simulink model "W14_Old_Town_cs"  (R2019a)
settings: Solver=ode5  StartTime=0.0  StopTime=inf  FixedStep=1/20  RelTol=1e-3
PreLoadFcn:
  | mbxruntime.callbacks.PreLoadFcn(bdroot);
PostLoadFcn:
  | mbxruntime.callbacks.PostLoadFcn(bdroot);
InitFcn:
  | mbxruntime.callbacks.InitFcn(bdroot);
StartFcn:
  | mbxruntime.callbacks.StartFcn(bdroot);
StopFcn:
  | mbxruntime.callbacks.StopFcn(bdroot);
model workspace: external: MAT-File .\W14_Old_Town_cs_hws.mat (data not in the file)
undefined symbols (not defined in the file or in its folder): DiscIntNeverNeededParam, InitImageOutputDir, mbxruntime, tabledata, W14_Old_Town_cs_420627b55bfa6657, W14_Old_Town_cs_65496e67f8744427, W14_Old_Town_cs_7675d4d8a4ff2559, W14_Old_Town_cs_7e35845ee4621ce0, W14_Old_Town_cs_873234be1b10e463, W14_Old_Town_cs_9ef39b80314364c8, W14_Old_Town_cs_a7463be4909f0caf, W14_Old_Town_cs_adbd81c42fc98a6f, W14_Old_Town_cs_Audi_A8_Sedan_1_Path_pathUniqueID, W14_Old_Town_cs_b1d069d1f3eacd72, W14_Old_Town_cs_Child_Regular_1_Path_pathUniqueID, W14_Old_Town_cs_Child_Regular_2_Path_pathUniqueID, W14_Old_Town_cs_Citroen_C3_Hatchback_1_Path_pathUniqueID, W14_Old_Town_cs_dbeb6fac3e8a4bef, W14_Old_Town_cs_fc5b0755bd4a98fc, W14_Old_Town_cs_Man_250_1_Path_pathUniqueID, W14_Old_Town_cs_Man_250_1_SpeedProfile_speedProfileUniqueID, W14_Old_Town_cs_Mazda_RX8_Coupe_1_Path_pathUniqueID
libraries: adeye_lib x38, simulink_extras x21, simulink x5, PreScanSimulinkLibrary x2, PreScanUsefulBlocks x1
(part 1 of 7)
CloseFcn:
  | mbxruntime.callbacks.CloseFcn(bdroot);
settings Model: Creator=PRESCAN  LastModifiedBy=adeye
settings DataIOCC: LimitDataPoints=on  SaveFormat=Array  SignalLoggingSaveFormat=ModelDataLogs  ReturnWorkspaceOutputs=off
settings OptimizationCC: DefaultParameterBehavior=Inlined  ExpressionDepthLimit=2147483647  InitFltsAndDblsToZero=on  LifeSpan=inf
settings DebuggingCC: SaveWithParameterizedLinksMsg=none  UnderspecifiedInitializationDetection=Classic  MergeDetectMultiDrivingBlocksExec=none  SignalResolutionControl=TryResolveAllWithWarning  MultiTaskDSMMsg=warning  MultiTaskCondExecSysMsg=none  FcnCallInpInsideContextMsg=warning  StateNameClashWarn=warning  SFUnexpectedBacktrackingDiag=warning  SFNoUnconditionalDefaultTransitionDiag=warning  SFExecutionAtInitializationDiag=none  ArithmeticOperatorsInVariantConditions=warning
settings HardwareCC: ProdBitPerPointer=32  ProdBitPerSizeT=32  ProdBitPerPtrDiffT=32  ProdLargestAtomicFloat=None  ProdIntDivRoundTo=Undefined  ProdEndianess=Unspecified  ProdWordSize=32  ProdHWDeviceType=32-bit Generic
settings ModelReferenceCC: UpdateModelReferenceTargets=IfOutOfDate  PropagateSignalLabelsOutOfModel=off
settings SFSimCC: SimUseLocalCustomCode=off  SimParseCustomCode=off
settings SFSimCC: SimCustomHeaderCode=|
  | #include "prescan.h"
  | #include "prescan_platform.h"
settings RTWCC: RTWUseLocalCustomCode=off
settings CodeAppCC: StateflowObjectComments=on
settings GRTTargetCC: TargetFcnLib=ansi_tfl_tmw.mat  TargetLangStandard=C89/C90 (ANSI)  GeneratePreprocessorConditionals=Disable all  CombineOutputUpdateFcns=off  GRTInterface=on
settings ConfigComp: CovMetricSettings=dw  CovHtmlReporting=on  CovSaveCumulativeToWorkspaceVar=on  CovSaveSingleToWorkspaceVar=on  CovExternalEMLEnable=off  CovSFcnEnable=off

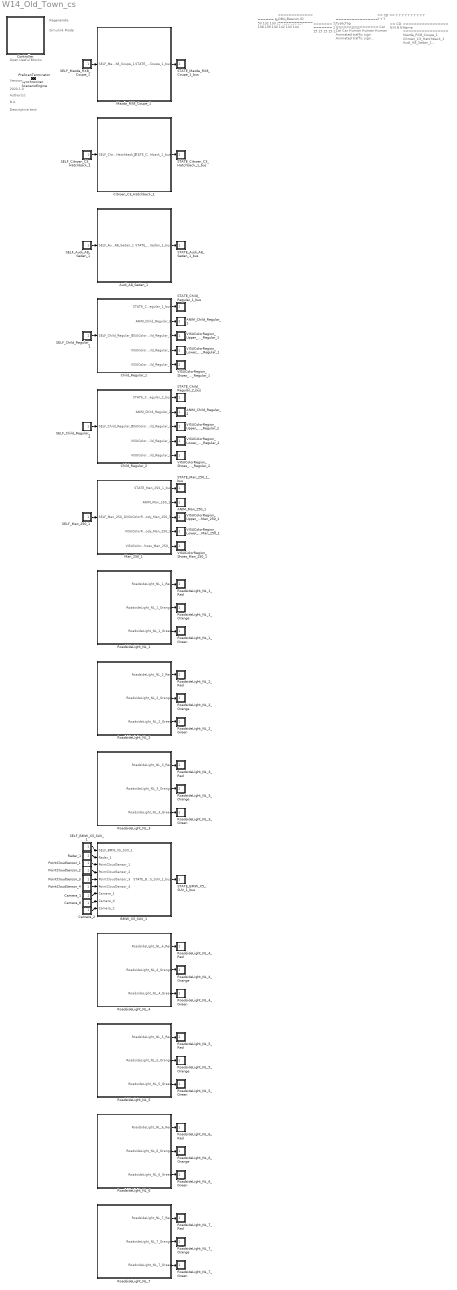
== system W14_Old_Town_cs ==
  note: Regenerate
  note: Simulink Mode
  note: Open Useful Blocks
  note: 2020.1.0
  note: Version:
  note: Author(s):
  note: N.A.
  note: Descriptive text:
  note: ======
      | Num ID
      | ======
      | 53
      | 132
      | 133
      | 134
      | 135
      | 136
      | 137
      | 138
      | 139
      | 140
      | 142
      | 143
      | 144
  note: =============
      | OBU-Beacon ID
      | =============
  note: =======
      | Type ID
      | =======
      | 1
      | 1
      | 1
      | 4
      | 4
      | 4
      | 15
      | 15
      | 15
      | 15
      | 15
      | 15
      | 15
  note: ================
      | Type Tag
      | ================
      | Car
      | Car
      | Car
      | Human
      | Human
      | Human
      | Animated traffic sign
      | Animated traffic sign
      | Animated traffic sign
      | Animated traffic sign
      | Animated traffic sign
      | Animated traffic sign
      | Animated traffic sign
  note: ==
      | SD
      | ==
      | Y
      | Y
      | Y
      | Y
      | Y
      | Y
      | Y
      | Y
      | Y
      | Y
      | Y
      | Y
      | Y
  note: ==
      | CD
      | ==
      | N
      | N
      | N
      | N
      | N
      | N
      | N
      | N
      | N
      | N
      | N
      | N
      | N
  note: =================
      | Name
      | =================
      | Mazda_RX8_Coupe_1
      | Citroen_C3_Hatchback_1
      | Audi_A8_Sedan_1
      | Child_Regular_1
      | Child_Regular_2
      | Man_250_1
      | RoadsideLight_NL_1
      | RoadsideLight_NL_2
      | RoadsideLight_NL_3
      | RoadsideLight_NL_4
      | RoadsideLight_NL_5
      | RoadsideLight_NL_6
      | RoadsideLight_NL_7
  ANIM_Child_Regular_1 : Subsystem  Tag=actuator/AnimationOutport  Priority=0  LoadFcn=load('PreScanAnimActuatorData.mat')  mask(PreScan Sink Block: State Animation){}
      mask help: The Human Animation port allows the human to walk, run or bend
      settings: OpenFcn=open_system([gcb '/Actuator'],'mask')
      mask Help: eval('openHelp(239)')
      mask Display: image(imread('HumanAnimated.jpg'))
  ANIM_Child_Regular_2 : Subsystem  Tag=actuator/AnimationOutport  Priority=0  LoadFcn=load('PreScanAnimActuatorData.mat')  mask(PreScan Sink Block: State Animation){}
      mask help: The Human Animation port allows the human to walk, run or bend
      settings: OpenFcn=open_system([gcb '/Actuator'],'mask')
      mask Help: eval('openHelp(239)')
      mask Display: image(imread('HumanAnimated.jpg'))
  ANIM_Man_250_1 : Subsystem  Tag=actuator/AnimationOutport  Priority=0  LoadFcn=load('PreScanAnimActuatorData.mat')  mask(PreScan Sink Block: State Animation){}
      mask help: The Human Animation port allows the human to walk, run or bend
      settings: OpenFcn=open_system([gcb '/Actuator'],'mask')
      mask Help: eval('openHelp(239)')
      mask Display: image(imread('HumanAnimated.jpg'))
  Audi_A8_Sedan_1 : Subsystem  Tag=WorldObjectSubSystem  InitFcn=UniqueId = '6579';
      mask init:
      | modelPath = GenericModelHelper.getGenericModelFilePath('ModelDepo','Vehicles\Audi_A8\Audi_A8.pgmb','e33fe1ddcf3e8ae97caccbc8f2fa74ac');imagePath = GenericModelHelper.getCompilationPicture(modelPath, 'Audi_A8_HighPoly.png');
      mask Display: image(imread(imagePath));color('white');text(0, 0, ' ID=133\n')
  BMW_X5_SUV_1 : Subsystem  Tag=WorldObjectSubSystem  InitFcn=|
      | UniqueId = '6361';
      | UniqueId = '6795';
      mask init:
      | modelPath = GenericModelHelper.getGenericModelFilePath('ModelDepo','Vehicles\BMW_X5\BMW_X5.pgmb','bfeb1c11467705ab888b3011684c848b');imagePath = GenericModelHelper.getCompilationPicture(modelPath, 'BMW_X5_HighPoly.png');
      mask Display: image(imread(imagePath));color('white');text(0, 0, ' ID=141\n')
  Camera_1 : Subsystem  Tag=sensor/Camera/CameraSensor  Priority=30  mask(PreScan Source Block: Camera Sensor){}
      mask help: The Camera Sensor provides a color or monochrome image.
      settings: OpenFcn=open_system([gcb '/Sensor'],'mask')
      mask Help: eval('openHelp(457)')
      mask Display: image(imread('CameraSensor.png'))
  Camera_2 : Subsystem  Tag=sensor/Camera/CameraSensor  Priority=30  mask(PreScan Source Block: Camera Sensor){}
      mask help: The Camera Sensor provides a color or monochrome image.
      settings: OpenFcn=open_system([gcb '/Sensor'],'mask')
      mask Help: eval('openHelp(457)')
      mask Display: image(imread('CameraSensor.png'))
  Camera_tl : Subsystem  Tag=sensor/Camera/CameraSensor  Priority=30  mask(PreScan Source Block: Camera Sensor){}
      mask help: The Camera Sensor provides a color or monochrome image.
      settings: OpenFcn=open_system([gcb '/Sensor'],'mask')
      mask Help: eval('openHelp(457)')
      mask Display: image(imread('CameraSensor.png'))
  Child_Regular_1 : Subsystem  Tag=WorldObjectSubSystem  InitFcn=UniqueId = '6584';
      mask init:
      | modelPath = GenericModelHelper.getGenericModelFilePath('ModelDepo','Humans\ChildRegular\Child_Regular.pgmb','0405fb6e1c51d7af34e60031bef9e83f');imagePath = GenericModelHelper.getCompilationPicture(modelPath, 'ChildRegular.png');
      mask Display: image(imread(imagePath));color('white');text(0, 0, ' ID=134\n')
  Child_Regular_2 : Subsystem  Tag=WorldObjectSubSystem  InitFcn=UniqueId = '6587';
      mask init: same as W14_Old_Town_cs/Child_Regular_1
      mask Display: image(imread(imagePath));color('white');text(0, 0, ' ID=135\n')
  Citroen_C3_Hatchback_1 : Subsystem  Tag=WorldObjectSubSystem  InitFcn=UniqueId = '6576';
      mask init:
      | modelPath = GenericModelHelper.getGenericModelFilePath('ModelDepo','Vehicles\Citroen_C3\Citroen_C3.pgmb','e804ced06d50dbfc6a2202ab3ad01b0c');imagePath = GenericModelHelper.getCompilationPicture(modelPath, 'Citroen_C3_HighPoly.png');
      mask Display: image(imread(imagePath));color('white');text(0, 0, ' ID=132\n')
  Controller : Subsystem  Description=8A3CD2955739A82C886C20AE3E253D78460D53180EE2C1B14CC08DF75A70BE77  Priority=-1  LoadFcn=load PreScanControllerData  mask(PreScan Simulation Controller){prescanversion='2020.1.0', ModelReferencing=off, TimeStep=1/20, ControlMode=0, PreScanExecutionMode=on, ControllerCount=0, ControllerIndex=0, ControllerOptions=''}
      mask prompts: prescanversion "PreScan Version"; ModelReferencing "Use Model Referencing"; TimeStep "Upload Period [s]"; ControlMode "Control Mode"; PreScanExecutionMode "Execution Mode"; ControllerCount "Controller Count"; ControllerIndex "Controller Index"; ControllerOptions "Controller Options"
      mask help:
      | Please do not remove this block from the compilation sheet,
      | as it connects the model to the PreScan environment.
      mask init:
      | model = bdroot(gcb);
      | ExperimentFile = mbxruntime.findExperimentFile(model,true); %relative path
      | 
      | [d1, d2, d3, prescandata] = prescan_Settings();
      | ModelDepo = fullfile(prescandata,'ModelDepo'); 
      | 
      | RTmode = mbxruntime.getRTMode(model);
      | 
      | SimulationMode = get_param(bdroot,'SimulationMode');
      | if strcmp(SimulationMode, 'rapid-accelerator')
      |     SimulationMode = 'external';
      | end
      | TargetName = get_param(bdroot,'SystemTargetFile');
      settings: ModelCloseFcn=assignin('base',['model_closed_' bdroot],true);
      mask Help: eval('openHelp(812)')
      mask Display: image(imread('prescanlogo.ico'))
  Man_250_1 : Subsystem  Tag=WorldObjectSubSystem  InitFcn=UniqueId = '6591';
      mask init:
      | modelPath = GenericModelHelper.getGenericModelFilePath('ModelDepo','Humans\Man_250\Man_250.pgmb','d552687b60780d871f7a0144e7f81878');imagePath = GenericModelHelper.getCompilationPicture(modelPath, 'Man_250.png');
      mask Display: image(imread(imagePath));color('white');text(0, 0, ' ID=136\n')
  Mazda_RX8_Coupe_1 : Subsystem  Tag=WorldObjectSubSystem  InitFcn=UniqueId = '6573';
      mask init:
      | modelPath = GenericModelHelper.getGenericModelFilePath('ModelDepo','Vehicles\Mazda_RX8\Mazda_RX8.pgmb','1e55a2e40efa576b7f4fb93bae35d605');imagePath = GenericModelHelper.getCompilationPicture(modelPath, 'Mazda_RX8_HighPoly.png');
      mask Display: image(imread(imagePath));color('white');text(0, 0, ' ID=53\n')
  PointCloudSensor_1 : Subsystem  Tag=sensor/PointCloudInport  Priority=30  mask(PreScan Source Block: Point Cloud Sensor){}
      mask help: The Point Cloud Sensor provides XYZ positions relative to the sensor
      settings: OpenFcn=open_system([gcb '/Sensor'],'mask')
      mask Help: eval('openHelp(6400)')
      mask Display: image(imread('PointCloudSensorSL.png'))
  PointCloudSensor_2 : Subsystem  Tag=sensor/PointCloudInport  Priority=30  mask(PreScan Source Block: Point Cloud Sensor){}
      mask help: The Point Cloud Sensor provides XYZ positions relative to the sensor
      settings: OpenFcn=open_system([gcb '/Sensor'],'mask')
      mask Help: eval('openHelp(6400)')
      mask Display: image(imread('PointCloudSensorSL.png'))
  PointCloudSensor_3 : Subsystem  Tag=sensor/PointCloudInport  Priority=30  mask(PreScan Source Block: Point Cloud Sensor){}
      mask help: The Point Cloud Sensor provides XYZ positions relative to the sensor
      settings: OpenFcn=open_system([gcb '/Sensor'],'mask')
      mask Help: eval('openHelp(6400)')
      mask Display: image(imread('PointCloudSensorSL.png'))
  PointCloudSensor_4 : Subsystem  Tag=sensor/PointCloudInport  Priority=30  mask(PreScan Source Block: Point Cloud Sensor){}
      mask help: The Point Cloud Sensor provides XYZ positions relative to the sensor
      settings: OpenFcn=open_system([gcb '/Sensor'],'mask')
      mask Help: eval('openHelp(6400)')
      mask Display: image(imread('PointCloudSensorSL.png'))
  PreScanTerminator : Subsystem  Tag=PreScanTerminator  Priority=999  LoadFcn=load PrescanTerminatorData  mask(PreScan Simulation Terminator){TimeStep=1/20}
      mask prompts: TimeStep "Upload Period [s]"
      mask help:
      | Please do not remove this block from the compilation sheet as it
      | connects the model to the PreScan environment.
      mask Help: eval('openHelp(812)')
      mask Display: image(imread('prescanlogo.ico'))
  Radar_1 : Subsystem  Tag=sensor/Radar  Priority=30  LoadFcn=load('PrescanScannerSensorData.mat');load('PrescanScannerSensorMessage.mat')  mask(PreScan Source Block: Radar Sensor){}
      mask help:
      | The Radar Sensor is a detailed sensor based on a physical radar
      | model that includes Antenna GAIN Maps (AGM) and atmospheric
      | attenuation.
      |
      | For more information, please click Help.
      settings: OpenFcn=open_system([gcb '/Sensor'],'mask')
      mask Help: eval('openHelp(1464)')
      mask Display: image(imread('Radar.png'))
  RoadsideLight_NL_1 : Subsystem  Tag=WorldObjectSubSystem  InitFcn=UniqueId = '6597';
      mask init:
      | modelPath = GenericModelHelper.getGenericModelFilePath('ModelDepo','AnimatedElements\TrafficLight_NL\Roadside\Roadside_NL.pgmb','2000fba5e1a6d0fba32e88146243c3cb');imagePath = GenericModelHelper.getCompilationPicture(modelPath, 'Roadside_NL.png');
      mask Display: image(imread(imagePath));color('white');text(0, 0, ' ID=137\n')
  RoadsideLight_NL_1_Green : Subsystem  Tag=actuator/Green  Priority=0  LoadFcn=load('PreScanVisuLightActuatorData');load('PrescanRPYData');load('PrescanXYZData');load('PreScanRGBData')  mask(PreScan Sink Block: VisuActiveLight){}
      mask help:
      | The VisuActiveLight block provides a way for detailed animation of Light Sources, such as the indicator, brake, fog and main lights of a vehicle, or a light post.
      |
      | For more information, please click Help.
      settings: OpenFcn=open_system([gcb '/Actuator'],'mask')
      mask Help: eval('openHelp(209)')
      mask Display: image(imread('HeadLight.png'))
  RoadsideLight_NL_1_Orange : Subsystem  Tag=actuator/Orange  Priority=0  LoadFcn=load('PreScanVisuLightActuatorData');load('PrescanRPYData');load('PrescanXYZData');load('PreScanRGBData')  mask(PreScan Sink Block: VisuActiveLight){}
      mask help:
      | The VisuActiveLight block provides a way for detailed animation of Light Sources, such as the indicator, brake, fog and main lights of a vehicle, or a light post.
      |
      | For more information, please click Help.
      settings: OpenFcn=open_system([gcb '/Actuator'],'mask')
      mask Help: eval('openHelp(209)')
      mask Display: image(imread('HeadLight.png'))
  RoadsideLight_NL_1_Red : Subsystem  Tag=actuator/Red  Priority=0  LoadFcn=load('PreScanVisuLightActuatorData');load('PrescanRPYData');load('PrescanXYZData');load('PreScanRGBData')  mask(PreScan Sink Block: VisuActiveLight){}
      mask help:
      | The VisuActiveLight block provides a way for detailed animation of Light Sources, such as the indicator, brake, fog and main lights of a vehicle, or a light post.
      |
      | For more information, please click Help.
      settings: OpenFcn=open_system([gcb '/Actuator'],'mask')
      mask Help: eval('openHelp(209)')
      mask Display: image(imread('HeadLight.png'))
  RoadsideLight_NL_2 : Subsystem  Tag=WorldObjectSubSystem  InitFcn=UniqueId = '6598';
      mask init: same as W14_Old_Town_cs/RoadsideLight_NL_1
      mask Display: image(imread(imagePath));color('white');text(0, 0, ' ID=138\n')
  RoadsideLight_NL_2_Green : Subsystem  Tag=actuator/Green  Priority=0  LoadFcn=load('PreScanVisuLightActuatorData');load('PrescanRPYData');load('PrescanXYZData');load('PreScanRGBData')  mask(PreScan Sink Block: VisuActiveLight){}
      mask help:
      | The VisuActiveLight block provides a way for detailed animation of Light Sources, such as the indicator, brake, fog and main lights of a vehicle, or a light post.
      |
      | For more information, please click Help.
      settings: OpenFcn=open_system([gcb '/Actuator'],'mask')
      mask Help: eval('openHelp(209)')
      mask Display: image(imread('HeadLight.png'))
  RoadsideLight_NL_2_Orange : Subsystem  Tag=actuator/Orange  Priority=0  LoadFcn=load('PreScanVisuLightActuatorData');load('PrescanRPYData');load('PrescanXYZData');load('PreScanRGBData')  mask(PreScan Sink Block: VisuActiveLight){}
      mask help:
      | The VisuActiveLight block provides a way for detailed animation of Light Sources, such as the indicator, brake, fog and main lights of a vehicle, or a light post.
      |
      | For more information, please click Help.
      settings: OpenFcn=open_system([gcb '/Actuator'],'mask')
      mask Help: eval('openHelp(209)')
      mask Display: image(imread('HeadLight.png'))
  RoadsideLight_NL_2_Red : Subsystem  Tag=actuator/Red  Priority=0  LoadFcn=load('PreScanVisuLightActuatorData');load('PrescanRPYData');load('PrescanXYZData');load('PreScanRGBData')  mask(PreScan Sink Block: VisuActiveLight){}
      mask help:
      | The VisuActiveLight block provides a way for detailed animation of Light Sources, such as the indicator, brake, fog and main lights of a vehicle, or a light post.
      |
      | For more information, please click Help.
      settings: OpenFcn=open_system([gcb '/Actuator'],'mask')
      mask Help: eval('openHelp(209)')
      mask Display: image(imread('HeadLight.png'))
  RoadsideLight_NL_3 : Subsystem  Tag=WorldObjectSubSystem  InitFcn=UniqueId = '6599';
      mask init: same as W14_Old_Town_cs/RoadsideLight_NL_1
      mask Display: image(imread(imagePath));color('white');text(0, 0, ' ID=139\n')
  RoadsideLight_NL_3_Green : Subsystem  Tag=actuator/Green  Priority=0  LoadFcn=load('PreScanVisuLightActuatorData');load('PrescanRPYData');load('PrescanXYZData');load('PreScanRGBData')  mask(PreScan Sink Block: VisuActiveLight){}
      mask help:
      | The VisuActiveLight block provides a way for detailed animation of Light Sources, such as the indicator, brake, fog and main lights of a vehicle, or a light post.
      |
      | For more information, please click Help.
      settings: OpenFcn=open_system([gcb '/Actuator'],'mask')
      mask Help: eval('openHelp(209)')
      mask Display: image(imread('HeadLight.png'))
  RoadsideLight_NL_3_Orange : Subsystem  Tag=actuator/Orange  Priority=0  LoadFcn=load('PreScanVisuLightActuatorData');load('PrescanRPYData');load('PrescanXYZData');load('PreScanRGBData')  mask(PreScan Sink Block: VisuActiveLight){}
      mask help:
      | The VisuActiveLight block provides a way for detailed animation of Light Sources, such as the indicator, brake, fog and main lights of a vehicle, or a light post.
      |
      | For more information, please click Help.
      settings: OpenFcn=open_system([gcb '/Actuator'],'mask')
      mask Help: eval('openHelp(209)')
      mask Display: image(imread('HeadLight.png'))
  RoadsideLight_NL_3_Red : Subsystem  Tag=actuator/Red  Priority=0  LoadFcn=load('PreScanVisuLightActuatorData');load('PrescanRPYData');load('PrescanXYZData');load('PreScanRGBData')  mask(PreScan Sink Block: VisuActiveLight){}
      mask help:
      | The VisuActiveLight block provides a way for detailed animation of Light Sources, such as the indicator, brake, fog and main lights of a vehicle, or a light post.
      |
      | For more information, please click Help.
      settings: OpenFcn=open_system([gcb '/Actuator'],'mask')
      mask Help: eval('openHelp(209)')
      mask Display: image(imread('HeadLight.png'))
  RoadsideLight_NL_4 : Subsystem  Tag=WorldObjectSubSystem  InitFcn=UniqueId = '6804';
      mask init: same as W14_Old_Town_cs/RoadsideLight_NL_1
      mask Display: image(imread(imagePath));color('white');text(0, 0, ' ID=140\n')
  RoadsideLight_NL_4_Green : Subsystem  Tag=actuator/Green  Priority=0  LoadFcn=load('PreScanVisuLightActuatorData');load('PrescanRPYData');load('PrescanXYZData');load('PreScanRGBData')  mask(PreScan Sink Block: VisuActiveLight){}
      mask help:
      | The VisuActiveLight block provides a way for detailed animation of Light Sources, such as the indicator, brake, fog and main lights of a vehicle, or a light post.
      |
      | For more information, please click Help.
      settings: OpenFcn=open_system([gcb '/Actuator'],'mask')
      mask Help: eval('openHelp(209)')
      mask Display: image(imread('HeadLight.png'))
  RoadsideLight_NL_4_Orange : Subsystem  Tag=actuator/Orange  Priority=0  LoadFcn=load('PreScanVisuLightActuatorData');load('PrescanRPYData');load('PrescanXYZData');load('PreScanRGBData')  mask(PreScan Sink Block: VisuActiveLight){}
      mask help:
      | The VisuActiveLight block provides a way for detailed animation of Light Sources, such as the indicator, brake, fog and main lights of a vehicle, or a light post.
      |
      | For more information, please click Help.
      settings: OpenFcn=open_system([gcb '/Actuator'],'mask')
      mask Help: eval('openHelp(209)')
      mask Display: image(imread('HeadLight.png'))
  RoadsideLight_NL_4_Red : Subsystem  Tag=actuator/Red  Priority=0  LoadFcn=load('PreScanVisuLightActuatorData');load('PrescanRPYData');load('PrescanXYZData');load('PreScanRGBData')  mask(PreScan Sink Block: VisuActiveLight){}
      mask help:
      | The VisuActiveLight block provides a way for detailed animation of Light Sources, such as the indicator, brake, fog and main lights of a vehicle, or a light post.
      |
      | For more information, please click Help.
      settings: OpenFcn=open_system([gcb '/Actuator'],'mask')
      mask Help: eval('openHelp(209)')
      mask Display: image(imread('HeadLight.png'))
  RoadsideLight_NL_5 : Subsystem  Tag=WorldObjectSubSystem  InitFcn=UniqueId = '6805';
      mask init: same as W14_Old_Town_cs/RoadsideLight_NL_1
      mask Display: image(imread(imagePath));color('white');text(0, 0, ' ID=142\n')
  RoadsideLight_NL_5_Green : Subsystem  Tag=actuator/Green  Priority=0  LoadFcn=load('PreScanVisuLightActuatorData');load('PrescanRPYData');load('PrescanXYZData');load('PreScanRGBData')  mask(PreScan Sink Block: VisuActiveLight){}
      mask help:
      | The VisuActiveLight block provides a way for detailed animation of Light Sources, such as the indicator, brake, fog and main lights of a vehicle, or a light post.
      |
      | For more information, please click Help.
      settings: OpenFcn=open_system([gcb '/Actuator'],'mask')
      mask Help: eval('openHelp(209)')
      mask Display: image(imread('HeadLight.png'))
  RoadsideLight_NL_5_Orange : Subsystem  Tag=actuator/Orange  Priority=0  LoadFcn=load('PreScanVisuLightActuatorData');load('PrescanRPYData');load('PrescanXYZData');load('PreScanRGBData')  mask(PreScan Sink Block: VisuActiveLight){}
      mask help:
      | The VisuActiveLight block provides a way for detailed animation of Light Sources, such as the indicator, brake, fog and main lights of a vehicle, or a light post.
      |
      | For more information, please click Help.
      settings: OpenFcn=open_system([gcb '/Actuator'],'mask')
      mask Help: eval('openHelp(209)')
      mask Display: image(imread('HeadLight.png'))
  RoadsideLight_NL_5_Red : Subsystem  Tag=actuator/Red  Priority=0  LoadFcn=load('PreScanVisuLightActuatorData');load('PrescanRPYData');load('PrescanXYZData');load('PreScanRGBData')  mask(PreScan Sink Block: VisuActiveLight){}
      mask help:
      | The VisuActiveLight block provides a way for detailed animation of Light Sources, such as the indicator, brake, fog and main lights of a vehicle, or a light post.
      |
      | For more information, please click Help.
      settings: OpenFcn=open_system([gcb '/Actuator'],'mask')
      mask Help: eval('openHelp(209)')
      mask Display: image(imread('HeadLight.png'))
  RoadsideLight_NL_6 : Subsystem  Tag=WorldObjectSubSystem  InitFcn=UniqueId = '6806';
      mask init: same as W14_Old_Town_cs/RoadsideLight_NL_1
      mask Display: image(imread(imagePath));color('white');text(0, 0, ' ID=143\n')
  RoadsideLight_NL_6_Green : Subsystem  Tag=actuator/Green  Priority=0  LoadFcn=load('PreScanVisuLightActuatorData');load('PrescanRPYData');load('PrescanXYZData');load('PreScanRGBData')  mask(PreScan Sink Block: VisuActiveLight){}
      mask help:
      | The VisuActiveLight block provides a way for detailed animation of Light Sources, such as the indicator, brake, fog and main lights of a vehicle, or a light post.
      |
      | For more information, please click Help.
      settings: OpenFcn=open_system([gcb '/Actuator'],'mask')
      mask Help: eval('openHelp(209)')
      mask Display: image(imread('HeadLight.png'))
  RoadsideLight_NL_6_Orange : Subsystem  Tag=actuator/Orange  Priority=0  LoadFcn=load('PreScanVisuLightActuatorData');load('PrescanRPYData');load('PrescanXYZData');load('PreScanRGBData')  mask(PreScan Sink Block: VisuActiveLight){}
      mask help:
      | The VisuActiveLight block provides a way for detailed animation of Light Sources, such as the indicator, brake, fog and main lights of a vehicle, or a light post.
      |
      | For more information, please click Help.
      settings: OpenFcn=open_system([gcb '/Actuator'],'mask')
      mask Help: eval('openHelp(209)')
      mask Display: image(imread('HeadLight.png'))
  RoadsideLight_NL_6_Red : Subsystem  Tag=actuator/Red  Priority=0  LoadFcn=load('PreScanVisuLightActuatorData');load('PrescanRPYData');load('PrescanXYZData');load('PreScanRGBData')  mask(PreScan Sink Block: VisuActiveLight){}
      mask help:
      | The VisuActiveLight block provides a way for detailed animation of Light Sources, such as the indicator, brake, fog and main lights of a vehicle, or a light post.
      |
      | For more information, please click Help.
      settings: OpenFcn=open_system([gcb '/Actuator'],'mask')
      mask Help: eval('openHelp(209)')
      mask Display: image(imread('HeadLight.png'))
  RoadsideLight_NL_7 : Subsystem  Tag=WorldObjectSubSystem  InitFcn=UniqueId = '6807';
      mask init: same as W14_Old_Town_cs/RoadsideLight_NL_1
      mask Display: image(imread(imagePath));color('white');text(0, 0, ' ID=144\n')
  RoadsideLight_NL_7_Green : Subsystem  Tag=actuator/Green  Priority=0  LoadFcn=load('PreScanVisuLightActuatorData');load('PrescanRPYData');load('PrescanXYZData');load('PreScanRGBData')  mask(PreScan Sink Block: VisuActiveLight){}
      mask help:
      | The VisuActiveLight block provides a way for detailed animation of Light Sources, such as the indicator, brake, fog and main lights of a vehicle, or a light post.
      |
      | For more information, please click Help.
      settings: OpenFcn=open_system([gcb '/Actuator'],'mask')
      mask Help: eval('openHelp(209)')
      mask Display: image(imread('HeadLight.png'))
  RoadsideLight_NL_7_Orange : Subsystem  Tag=actuator/Orange  Priority=0  LoadFcn=load('PreScanVisuLightActuatorData');load('PrescanRPYData');load('PrescanXYZData');load('PreScanRGBData')  mask(PreScan Sink Block: VisuActiveLight){}
      mask help:
      | The VisuActiveLight block provides a way for detailed animation of Light Sources, such as the indicator, brake, fog and main lights of a vehicle, or a light post.
      |
      | For more information, please click Help.
      settings: OpenFcn=open_system([gcb '/Actuator'],'mask')
      mask Help: eval('openHelp(209)')
      mask Display: image(imread('HeadLight.png'))
  RoadsideLight_NL_7_Red : Subsystem  Tag=actuator/Red  Priority=0  LoadFcn=load('PreScanVisuLightActuatorData');load('PrescanRPYData');load('PrescanXYZData');load('PreScanRGBData')  mask(PreScan Sink Block: VisuActiveLight){}
      mask help:
      | The VisuActiveLight block provides a way for detailed animation of Light Sources, such as the indicator, brake, fog and main lights of a vehicle, or a light post.
      |
      | For more information, please click Help.
      settings: OpenFcn=open_system([gcb '/Actuator'],'mask')
      mask Help: eval('openHelp(209)')
      mask Display: image(imread('HeadLight.png'))
  SELF_Audi_A8_Sedan_1 : Subsystem  Tag=sensor/SelfPort  Priority=30  LoadFcn=load('PreScanSelfSensorData.mat')  mask(PreScan Source Block: SELF){}
      mask help:
      | The SELF port shows (state) information of the actor itself. The outputs are position in the experiment's axis system and the GPS coordinates, and the object's absolute velocity and compass heading.
      |
      | For more information, please click Help.
      settings: OpenFcn=open_system([gcb '/Sensor'],'mask')
      mask Help: eval('openHelp(462)')
      mask Display: image(imread('GPS.png'))
  SELF_BMW_X5_SUV_1 : Subsystem  Tag=sensor/SelfPort  Priority=30  LoadFcn=load('PreScanSelfSensorData.mat')  mask(PreScan Source Block: SELF){}
      mask help:
      | The SELF port shows (state) information of the actor itself. The outputs are position in the experiment's axis system and the GPS coordinates, and the object's absolute velocity and compass heading.
      |
      | For more information, please click Help.
      settings: OpenFcn=open_system([gcb '/Sensor'],'mask')
      mask Help: eval('openHelp(462)')
      mask Display: image(imread('GPS.png'))
  SELF_Child_Regular_1 : Subsystem  Tag=sensor/SelfPort  Priority=30  LoadFcn=load('PreScanSelfSensorData.mat')  mask(PreScan Source Block: SELF){}
      mask help:
      | The SELF port shows (state) information of the actor itself. The outputs are position in the experiment's axis system and the GPS coordinates, and the object's absolute velocity and compass heading.
      |
      | For more information, please click Help.
      settings: OpenFcn=open_system([gcb '/Sensor'],'mask')
      mask Help: eval('openHelp(462)')
      mask Display: image(imread('GPS.png'))
  SELF_Child_Regular_2 : Subsystem  Tag=sensor/SelfPort  Priority=30  LoadFcn=load('PreScanSelfSensorData.mat')  mask(PreScan Source Block: SELF){}
      mask help:
      | The SELF port shows (state) information of the actor itself. The outputs are position in the experiment's axis system and the GPS coordinates, and the object's absolute velocity and compass heading.
      |
      | For more information, please click Help.
      settings: OpenFcn=open_system([gcb '/Sensor'],'mask')
      mask Help: eval('openHelp(462)')
      mask Display: image(imread('GPS.png'))
  SELF_Citroen_C3_Hatchback_1 : Subsystem  Tag=sensor/SelfPort  Priority=30  LoadFcn=load('PreScanSelfSensorData.mat')  mask(PreScan Source Block: SELF){}
      mask help:
      | The SELF port shows (state) information of the actor itself. The outputs are position in the experiment's axis system and the GPS coordinates, and the object's absolute velocity and compass heading.
      |
      | For more information, please click Help.
      settings: OpenFcn=open_system([gcb '/Sensor'],'mask')
      mask Help: eval('openHelp(462)')
      mask Display: image(imread('GPS.png'))
  SELF_Man_250_1 : Subsystem  Tag=sensor/SelfPort  Priority=30  LoadFcn=load('PreScanSelfSensorData.mat')  mask(PreScan Source Block: SELF){}
      mask help:
      | The SELF port shows (state) information of the actor itself. The outputs are position in the experiment's axis system and the GPS coordinates, and the object's absolute velocity and compass heading.
      |
      | For more information, please click Help.
      settings: OpenFcn=open_system([gcb '/Sensor'],'mask')
      mask Help: eval('openHelp(462)')
      mask Display: image(imread('GPS.png'))
  SELF_Mazda_RX8_Coupe_1 : Subsystem  Tag=sensor/SelfPort  Priority=30  LoadFcn=load('PreScanSelfSensorData.mat')  mask(PreScan Source Block: SELF){}
      mask help:
      | The SELF port shows (state) information of the actor itself. The outputs are position in the experiment's axis system and the GPS coordinates, and the object's absolute velocity and compass heading.
      |
      | For more information, please click Help.
      settings: OpenFcn=open_system([gcb '/Sensor'],'mask')
      mask Help: eval('openHelp(462)')
      mask Display: image(imread('GPS.png'))
  STATE_Audi_A8_Sedan_1_bus : Subsystem  Tag=actuator/StatePort  Priority=0  LoadFcn=load('PreScanStateActuatorData.mat')  mask(PreScan Sink Block: State){}
      mask help:
      | The Actor State contains a vector signal of size (9x1), containing the following signals:
      |
      | -  Position    	(x,y,z)             	[m]
      | -  Velocity    	(vx,vy,vz)         	[m/s]
      | -  Angles       	(Roll, Pitch, Yaw)	[rad]
      |
      | The Actor state is defined in the global axis system.
      | The state is superponed on the Initial position defined in the GUI.
      |
      | For more information, please click Help.
      settings: OpenFcn=open_system([gcb '/Actuator'],'mask')
      mask Help: eval('openHelp(222)')
      mask Display: image(imread('State.png'))
  STATE_BMW_X5_SUV_1_bus : Subsystem  Tag=actuator/StatePort  Priority=0  LoadFcn=load('PreScanStateActuatorData.mat')  mask(PreScan Sink Block: State){}
      mask help:
      | The Actor State contains a vector signal of size (9x1), containing the following signals:
      |
      | -  Position    	(x,y,z)             	[m]
      | -  Velocity    	(vx,vy,vz)         	[m/s]
      | -  Angles       	(Roll, Pitch, Yaw)	[rad]
      |
      | The Actor state is defined in the global axis system.
      | The state is superponed on the Initial position defined in the GUI.
      |
      | For more information, please click Help.
      settings: OpenFcn=open_system([gcb '/Actuator'],'mask')
      mask Help: eval('openHelp(222)')
      mask Display: image(imread('State.png'))
  STATE_Child_Regular_1_bus : Subsystem  Tag=actuator/StatePort  Priority=0  LoadFcn=load('PreScanStateActuatorData.mat')  mask(PreScan Sink Block: State){}
      mask help:
      | The Actor State contains a vector signal of size (9x1), containing the following signals:
      |
      | -  Position    	(x,y,z)             	[m]
      | -  Velocity    	(vx,vy,vz)         	[m/s]
      | -  Angles       	(Roll, Pitch, Yaw)	[rad]
      |
      | The Actor state is defined in the global axis system.
      | The state is superponed on the Initial position defined in the GUI.
      |
      | For more information, please click Help.
      settings: OpenFcn=open_system([gcb '/Actuator'],'mask')
      mask Help: eval('openHelp(222)')
      mask Display: image(imread('State.png'))
  STATE_Child_Regular_2_bus : Subsystem  Tag=actuator/StatePort  Priority=0  LoadFcn=load('PreScanStateActuatorData.mat')  mask(PreScan Sink Block: State){}
      mask help:
      | The Actor State contains a vector signal of size (9x1), containing the following signals:
      |
      | -  Position    	(x,y,z)             	[m]
      | -  Velocity    	(vx,vy,vz)         	[m/s]
      | -  Angles       	(Roll, Pitch, Yaw)	[rad]
      |
      | The Actor state is defined in the global axis system.
      | The state is superponed on the Initial position defined in the GUI.
      |
      | For more information, please click Help.
      settings: OpenFcn=open_system([gcb '/Actuator'],'mask')
      mask Help: eval('openHelp(222)')
      mask Display: image(imread('State.png'))
  STATE_Citroen_C3_Hatchback_1_bus : Subsystem  Tag=actuator/StatePort  Priority=0  LoadFcn=load('PreScanStateActuatorData.mat')  mask(PreScan Sink Block: State){}
      mask help:
      | The Actor State contains a vector signal of size (9x1), containing the following signals:
      |
      | -  Position    	(x,y,z)             	[m]
      | -  Velocity    	(vx,vy,vz)         	[m/s]
      | -  Angles       	(Roll, Pitch, Yaw)	[rad]
      |
      | The Actor state is defined in the global axis system.
      | The state is superponed on the Initial position defined in the GUI.
      |
      | For more information, please click Help.
      settings: OpenFcn=open_system([gcb '/Actuator'],'mask')
      mask Help: eval('openHelp(222)')
      mask Display: image(imread('State.png'))
  STATE_Man_250_1_bus : Subsystem  Tag=actuator/StatePort  Priority=0  LoadFcn=load('PreScanStateActuatorData.mat')  mask(PreScan Sink Block: State){}
      mask help:
      | The Actor State contains a vector signal of size (9x1), containing the following signals:
      |
      | -  Position    	(x,y,z)             	[m]
      | -  Velocity    	(vx,vy,vz)         	[m/s]
      | -  Angles       	(Roll, Pitch, Yaw)	[rad]
      |
      | The Actor state is defined in the global axis system.
      | The state is superponed on the Initial position defined in the GUI.
      |
      | For more information, please click Help.
      settings: OpenFcn=open_system([gcb '/Actuator'],'mask')
      mask Help: eval('openHelp(222)')
      mask Display: image(imread('State.png'))
  STATE_Mazda_RX8_Coupe_1_bus : Subsystem  Tag=actuator/StatePort  Priority=0  LoadFcn=load('PreScanStateActuatorData.mat')  mask(PreScan Sink Block: State){}
      mask help:
      | The Actor State contains a vector signal of size (9x1), containing the following signals:
      |
      | -  Position    	(x,y,z)             	[m]
      | -  Velocity    	(vx,vy,vz)         	[m/s]
      | -  Angles       	(Roll, Pitch, Yaw)	[rad]
      |
      | The Actor state is defined in the global axis system.
      | The state is superponed on the Initial position defined in the GUI.
      |
      | For more information, please click Help.
      settings: OpenFcn=open_system([gcb '/Actuator'],'mask')
      mask Help: eval('openHelp(222)')
      mask Display: image(imread('State.png'))
  ScenarioEngine : Subsystem  Tag=PreScanOpenScenarioBlock  Priority=10  LoadFcn=load PrescanSynchronizeData  mask(PreScan Simulation Core Block){TimeStep=1/20}
      mask prompts: TimeStep "Timestep [s]"
      mask help:
      | Please do not remove this block from the PreScan compilation sheet,
      | as it contains essential configuration parameters for a PreScan simulation.
      settings: DeleteFcn=PreScanBlockDeleteFcn;
      mask Display: image(imread('prescanlogo.ico'))
  Synchronizer : Subsystem  Tag=PreScanSynchronizer  Priority=20  LoadFcn=load PrescanSynchronizeData  mask(PreScan Simulation Core Block){TimeStep=1/20}
      mask prompts: TimeStep "Timestep [s]"
      mask help:
      | Please do not remove this block from the PreScan compilation sheet,
      | as it contains essential configuration parameters for a PreScan simulation.
      settings: DeleteFcn=PreScanBlockDeleteFcn;
      mask Display: image(imread('prescanlogo.ico'))
  VISUColorRegion_Lower_Body_Child_Regular_1 : Subsystem  Tag=actuator/ColorRegion  Priority=0  LoadFcn=load('PrescanColorData')  mask(PreScan Sink Block: VisuTextureColor){}
      mask help:
      | The VisuTextureColor block provides a way to adapt the color of a vehicle.
      |
      | For more information, please click Help.
      settings: OpenFcn=open_system([gcb '/Actuator'],'mask')
      mask Help: eval('openHelp(230)')
      mask Display: image(imread('TextureColor.png'))
  VISUColorRegion_Lower_Body_Child_Regular_2 : Subsystem  Tag=actuator/ColorRegion  Priority=0  LoadFcn=load('PrescanColorData')  mask(PreScan Sink Block: VisuTextureColor){}
      mask help:
      | The VisuTextureColor block provides a way to adapt the color of a vehicle.
      |
      | For more information, please click Help.
      settings: OpenFcn=open_system([gcb '/Actuator'],'mask')
      mask Help: eval('openHelp(230)')
      mask Display: image(imread('TextureColor.png'))
  VISUColorRegion_Lower_Body_Man_250_1 : Subsystem  Tag=actuator/ColorRegion  Priority=0  LoadFcn=load('PrescanColorData')  mask(PreScan Sink Block: VisuTextureColor){}
      mask help:
      | The VisuTextureColor block provides a way to adapt the color of a vehicle.
      |
      | For more information, please click Help.
      settings: OpenFcn=open_system([gcb '/Actuator'],'mask')
      mask Help: eval('openHelp(230)')
      mask Display: image(imread('TextureColor.png'))
  VISUColorRegion_Shoes_Child_Regular_1 : Subsystem  Tag=actuator/ColorRegion  Priority=0  LoadFcn=load('PrescanColorData')  mask(PreScan Sink Block: VisuTextureColor){}
      mask help:
      | The VisuTextureColor block provides a way to adapt the color of a vehicle.
      |
      | For more information, please click Help.
      settings: OpenFcn=open_system([gcb '/Actuator'],'mask')
      mask Help: eval('openHelp(230)')
      mask Display: image(imread('TextureColor.png'))
  VISUColorRegion_Shoes_Child_Regular_2 : Subsystem  Tag=actuator/ColorRegion  Priority=0  LoadFcn=load('PrescanColorData')  mask(PreScan Sink Block: VisuTextureColor){}
      mask help:
      | The VisuTextureColor block provides a way to adapt the color of a vehicle.
      |
      | For more information, please click Help.
      settings: OpenFcn=open_system([gcb '/Actuator'],'mask')
      mask Help: eval('openHelp(230)')
      mask Display: image(imread('TextureColor.png'))
  VISUColorRegion_Shoes_Man_250_1 : Subsystem  Tag=actuator/ColorRegion  Priority=0  LoadFcn=load('PrescanColorData')  mask(PreScan Sink Block: VisuTextureColor){}
      mask help:
      | The VisuTextureColor block provides a way to adapt the color of a vehicle.
      |
      | For more information, please click Help.
      settings: OpenFcn=open_system([gcb '/Actuator'],'mask')
      mask Help: eval('openHelp(230)')
      mask Display: image(imread('TextureColor.png'))
  VISUColorRegion_Upper_Body_Child_Regular_1 : Subsystem  Tag=actuator/ColorRegion  Priority=0  LoadFcn=load('PrescanColorData')  mask(PreScan Sink Block: VisuTextureColor){}
      mask help:
      | The VisuTextureColor block provides a way to adapt the color of a vehicle.
      |
      | For more information, please click Help.
      settings: OpenFcn=open_system([gcb '/Actuator'],'mask')
      mask Help: eval('openHelp(230)')
      mask Display: image(imread('TextureColor.png'))
  VISUColorRegion_Upper_Body_Child_Regular_2 : Subsystem  Tag=actuator/ColorRegion  Priority=0  LoadFcn=load('PrescanColorData')  mask(PreScan Sink Block: VisuTextureColor){}
      mask help:
      | The VisuTextureColor block provides a way to adapt the color of a vehicle.
      |
      | For more information, please click Help.
      settings: OpenFcn=open_system([gcb '/Actuator'],'mask')
      mask Help: eval('openHelp(230)')
      mask Display: image(imread('TextureColor.png'))
  VISUColorRegion_Upper_Body_Man_250_1 : Subsystem  Tag=actuator/ColorRegion  Priority=0  LoadFcn=load('PrescanColorData')  mask(PreScan Sink Block: VisuTextureColor){}
      mask help:
      | The VisuTextureColor block provides a way to adapt the color of a vehicle.
      |
      | For more information, please click Help.
      settings: OpenFcn=open_system([gcb '/Actuator'],'mask')
      mask Help: eval('openHelp(230)')
      mask Display: image(imread('TextureColor.png'))
  wires:
  Mazda_RX8_Coupe_1/1(STATE_Mazda_RX8_Coupe_1_bus) -> STATE_Mazda_RX8_Coupe_1_bus/1(STATE_Mazda_RX8_Coupe_1_bus)
  SELF_Mazda_RX8_Coupe_1/1(SELF_Mazda_RX8_Coupe_1) -> Mazda_RX8_Coupe_1/1(SELF_Mazda_RX8_Coupe_1)
  Citroen_C3_Hatchback_1/1(STATE_Citroen_C3_Hatchback_1_bus) -> STATE_Citroen_C3_Hatchback_1_bus/1(STATE_Citroen_C3_Hatchback_1_bus)
  SELF_Citroen_C3_Hatchback_1/1(SELF_Citroen_C3_Hatchback_1) -> Citroen_C3_Hatchback_1/1(SELF_Citroen_C3_Hatchback_1)
  Audi_A8_Sedan_1/1(STATE_Audi_A8_Sedan_1_bus) -> STATE_Audi_A8_Sedan_1_bus/1(STATE_Audi_A8_Sedan_1_bus)
  SELF_Audi_A8_Sedan_1/1(SELF_Audi_A8_Sedan_1) -> Audi_A8_Sedan_1/1(SELF_Audi_A8_Sedan_1)
  Child_Regular_1/1(STATE_Child_Regular_1_bus) -> STATE_Child_Regular_1_bus/1(STATE_Child_Regular_1_bus)
  Child_Regular_1/2(ANIM_Child_Regular_1) -> ANIM_Child_Regular_1/1(ANIM_Child_Regular_1)
  SELF_Child_Regular_1/1(SELF_Child_Regular_1) -> Child_Regular_1/1(SELF_Child_Regular_1)
  Child_Regular_1/3(VISUColorRegion_Upper_Body_Child_Regular_1) -> VISUColorRegion_Upper_Body_Child_Regular_1/1(VISUColorRegion_Upper_Body_Child_Regular_1)
  Child_Regular_1/4(VISUColorRegion_Lower_Body_Child_Regular_1) -> VISUColorRegion_Lower_Body_Child_Regular_1/1(VISUColorRegion_Lower_Body_Child_Regular_1)
  Child_Regular_1/5(VISUColorRegion_Shoes_Child_Regular_1) -> VISUColorRegion_Shoes_Child_Regular_1/1(VISUColorRegion_Shoes_Child_Regular_1)
  Child_Regular_2/1(STATE_Child_Regular_2_bus) -> STATE_Child_Regular_2_bus/1(STATE_Child_Regular_2_bus)
  Child_Regular_2/2(ANIM_Child_Regular_2) -> ANIM_Child_Regular_2/1(ANIM_Child_Regular_2)
  SELF_Child_Regular_2/1(SELF_Child_Regular_2) -> Child_Regular_2/1(SELF_Child_Regular_2)
  Child_Regular_2/3(VISUColorRegion_Upper_Body_Child_Regular_2) -> VISUColorRegion_Upper_Body_Child_Regular_2/1(VISUColorRegion_Upper_Body_Child_Regular_2)
  Child_Regular_2/4(VISUColorRegion_Lower_Body_Child_Regular_2) -> VISUColorRegion_Lower_Body_Child_Regular_2/1(VISUColorRegion_Lower_Body_Child_Regular_2)
  Child_Regular_2/5(VISUColorRegion_Shoes_Child_Regular_2) -> VISUColorRegion_Shoes_Child_Regular_2/1(VISUColorRegion_Shoes_Child_Regular_2)
  Man_250_1/1(STATE_Man_250_1_bus) -> STATE_Man_250_1_bus/1(STATE_Man_250_1_bus)
  Man_250_1/2(ANIM_Man_250_1) -> ANIM_Man_250_1/1(ANIM_Man_250_1)
  SELF_Man_250_1/1(SELF_Man_250_1) -> Man_250_1/1(SELF_Man_250_1)
  Man_250_1/3(VISUColorRegion_Upper_Body_Man_250_1) -> VISUColorRegion_Upper_Body_Man_250_1/1(VISUColorRegion_Upper_Body_Man_250_1)
  Man_250_1/4(VISUColorRegion_Lower_Body_Man_250_1) -> VISUColorRegion_Lower_Body_Man_250_1/1(VISUColorRegion_Lower_Body_Man_250_1)
  Man_250_1/5(VISUColorRegion_Shoes_Man_250_1) -> VISUColorRegion_Shoes_Man_250_1/1(VISUColorRegion_Shoes_Man_250_1)
  RoadsideLight_NL_1/1(RoadsideLight_NL_1_Red) -> RoadsideLight_NL_1_Red/1(RoadsideLight_NL_1_Red)
  RoadsideLight_NL_1/2(RoadsideLight_NL_1_Orange) -> RoadsideLight_NL_1_Orange/1(RoadsideLight_NL_1_Orange)
  RoadsideLight_NL_1/3(RoadsideLight_NL_1_Green) -> RoadsideLight_NL_1_Green/1(RoadsideLight_NL_1_Green)
  RoadsideLight_NL_2/1(RoadsideLight_NL_2_Red) -> RoadsideLight_NL_2_Red/1(RoadsideLight_NL_2_Red)
  RoadsideLight_NL_2/2(RoadsideLight_NL_2_Orange) -> RoadsideLight_NL_2_Orange/1(RoadsideLight_NL_2_Orange)
  RoadsideLight_NL_2/3(RoadsideLight_NL_2_Green) -> RoadsideLight_NL_2_Green/1(RoadsideLight_NL_2_Green)
  RoadsideLight_NL_3/1(RoadsideLight_NL_3_Red) -> RoadsideLight_NL_3_Red/1(RoadsideLight_NL_3_Red)
  RoadsideLight_NL_3/2(RoadsideLight_NL_3_Orange) -> RoadsideLight_NL_3_Orange/1(RoadsideLight_NL_3_Orange)
  RoadsideLight_NL_3/3(RoadsideLight_NL_3_Green) -> RoadsideLight_NL_3_Green/1(RoadsideLight_NL_3_Green)
  BMW_X5_SUV_1/1(STATE_BMW_X5_SUV_1_bus) -> STATE_BMW_X5_SUV_1_bus/1(STATE_BMW_X5_SUV_1_bus)
  SELF_BMW_X5_SUV_1/1(SELF_BMW_X5_SUV_1) -> BMW_X5_SUV_1/1(SELF_BMW_X5_SUV_1)
  Radar_1/1(Radar_1) -> BMW_X5_SUV_1/2(Radar_1)
  PointCloudSensor_1/1(PointCloudSensor_1) -> BMW_X5_SUV_1/3(PointCloudSensor_1)
  PointCloudSensor_2/1(PointCloudSensor_2) -> BMW_X5_SUV_1/4(PointCloudSensor_2)
  PointCloudSensor_3/1(PointCloudSensor_3) -> BMW_X5_SUV_1/5(PointCloudSensor_3)
  PointCloudSensor_4/1(PointCloudSensor_4) -> BMW_X5_SUV_1/6(PointCloudSensor_4)
  Camera_1/1(Camera_1) -> BMW_X5_SUV_1/7(Camera_1)
  Camera_tl/1(Camera_tl) -> BMW_X5_SUV_1/8(Camera_tl)
  Camera_2/1(Camera_2) -> BMW_X5_SUV_1/9(Camera_2)
  RoadsideLight_NL_4/1(RoadsideLight_NL_4_Red) -> RoadsideLight_NL_4_Red/1(RoadsideLight_NL_4_Red)
  RoadsideLight_NL_4/2(RoadsideLight_NL_4_Orange) -> RoadsideLight_NL_4_Orange/1(RoadsideLight_NL_4_Orange)
  RoadsideLight_NL_4/3(RoadsideLight_NL_4_Green) -> RoadsideLight_NL_4_Green/1(RoadsideLight_NL_4_Green)
  RoadsideLight_NL_5/1(RoadsideLight_NL_5_Red) -> RoadsideLight_NL_5_Red/1(RoadsideLight_NL_5_Red)
  RoadsideLight_NL_5/2(RoadsideLight_NL_5_Orange) -> RoadsideLight_NL_5_Orange/1(RoadsideLight_NL_5_Orange)
  RoadsideLight_NL_5/3(RoadsideLight_NL_5_Green) -> RoadsideLight_NL_5_Green/1(RoadsideLight_NL_5_Green)
  RoadsideLight_NL_6/1(RoadsideLight_NL_6_Red) -> RoadsideLight_NL_6_Red/1(RoadsideLight_NL_6_Red)
  RoadsideLight_NL_6/2(RoadsideLight_NL_6_Orange) -> RoadsideLight_NL_6_Orange/1(RoadsideLight_NL_6_Orange)
  RoadsideLight_NL_6/3(RoadsideLight_NL_6_Green) -> RoadsideLight_NL_6_Green/1(RoadsideLight_NL_6_Green)
  RoadsideLight_NL_7/1(RoadsideLight_NL_7_Red) -> RoadsideLight_NL_7_Red/1(RoadsideLight_NL_7_Red)
  RoadsideLight_NL_7/2(RoadsideLight_NL_7_Orange) -> RoadsideLight_NL_7_Orange/1(RoadsideLight_NL_7_Orange)
  RoadsideLight_NL_7/3(RoadsideLight_NL_7_Green) -> RoadsideLight_NL_7_Green/1(RoadsideLight_NL_7_Green)

== system W14_Old_Town_cs/ANIM_Child_Regular_1 ==
  ANIM_Child_Regular_1 : Inport  Tag=inport/AnimationOutport  OutDataTypeStr=Bus: PRESCAN_ANIMACTUATORDATA  PortDimensions=1  SampleTime=1/20  BusOutputAsStruct=on
  Actuator : S-Function  FunctionName=sfun_AnimActuator  Parameters=UniqueID, TimeStep  SFunctionDeploymentMode=off  EnableBusSupport=off  mask(PreScan Sink Block: State Animation){UniqueID=6584, TimeStep=1/20}
      mask prompts: UniqueID "Auto-Assigned: Unique ID"; TimeStep "Auto-Assigned: Upload Period [s]"
      mask help: The Human Animation port allows the human to walk, run or bend
      mask Help: eval('openHelp(239)')
      mask Display: image(imread('HumanAnimated.jpg'))
  wires:
  ANIM_Child_Regular_1/1 -> Actuator/1

== system W14_Old_Town_cs/ANIM_Child_Regular_2 ==
  ANIM_Child_Regular_2 : Inport  Tag=inport/AnimationOutport  OutDataTypeStr=Bus: PRESCAN_ANIMACTUATORDATA  PortDimensions=1  SampleTime=1/20  BusOutputAsStruct=on
  Actuator : S-Function  FunctionName=sfun_AnimActuator  Parameters=UniqueID, TimeStep  SFunctionDeploymentMode=off  EnableBusSupport=off  mask(PreScan Sink Block: State Animation){UniqueID=6587, TimeStep=1/20}
      mask prompts: UniqueID "Auto-Assigned: Unique ID"; TimeStep "Auto-Assigned: Upload Period [s]"
      mask help: The Human Animation port allows the human to walk, run or bend
      mask Help: eval('openHelp(239)')
      mask Display: image(imread('HumanAnimated.jpg'))
  wires:
  ANIM_Child_Regular_2/1 -> Actuator/1

== system W14_Old_Town_cs/ANIM_Man_250_1 ==
  ANIM_Man_250_1 : Inport  Tag=inport/AnimationOutport  OutDataTypeStr=Bus: PRESCAN_ANIMACTUATORDATA  PortDimensions=1  SampleTime=1/20  BusOutputAsStruct=on
  Actuator : S-Function  FunctionName=sfun_AnimActuator  Parameters=UniqueID, TimeStep  SFunctionDeploymentMode=off  EnableBusSupport=off  mask(PreScan Sink Block: State Animation){UniqueID=6591, TimeStep=1/20}
      mask prompts: UniqueID "Auto-Assigned: Unique ID"; TimeStep "Auto-Assigned: Upload Period [s]"
      mask help: The Human Animation port allows the human to walk, run or bend
      mask Help: eval('openHelp(239)')
      mask Display: image(imread('HumanAnimated.jpg'))
  wires:
  ANIM_Man_250_1/1 -> Actuator/1
